simulink model "Plant"  (R2023a)
settings: Solver=VariableStepAuto  StartTime=0.0  StopTime=20  RelTol=1e-3
libraries: slpidlib x2
settings Model: Creator=abhi2  LastModifiedBy=abhi2
settings DebuggingCC: AlgebraicLoopMsg=none

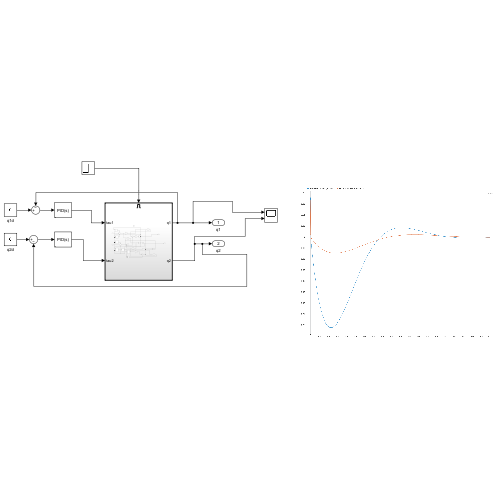
[thumbnail: Simulink's stored preview of the top-level diagram]
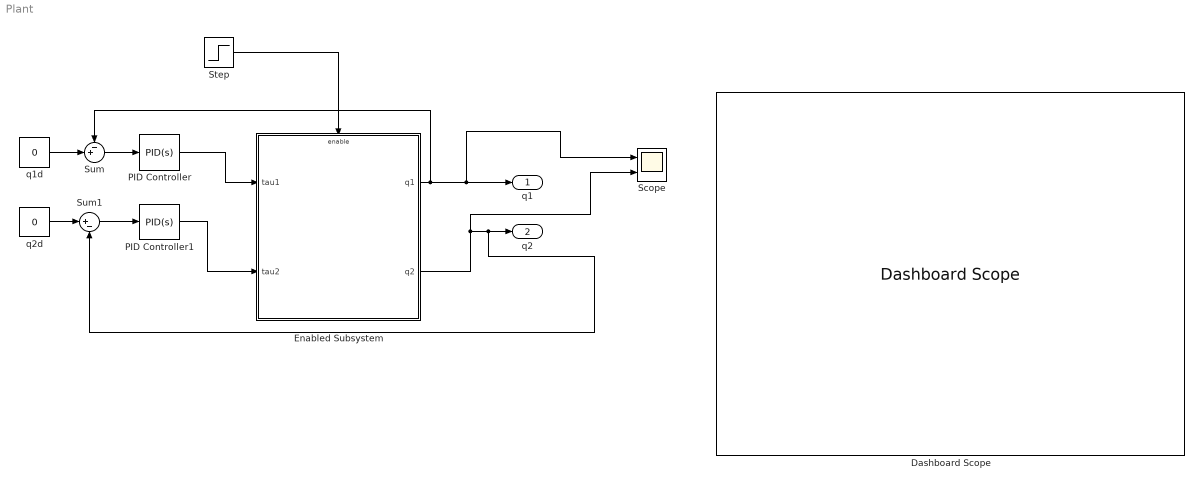
== system Plant ==
  Dashboard Scope : DashboardScope  Ymin=-0.8  Ymax=0.15
  Enabled Subsystem : Subsystem  TreatAsAtomicUnit=on
  PID Controller : slpidlib/PID Controller  Controller=PID  Form=Parallel  TimeDomain=Continuous-time  UseExternalTs=off  SampleTime=-1  IntegratorMethod=Forward Euler  FilterMethod=Forward Euler  ControllerParametersSource=internal  P=80  I=70  UseKiTs=off  D=70  N=1000000  UseFilter=on  TunerSelectOption=Transfer Function Based (PID Tuner App)  InitialConditionSource=internal  InitialConditionForIntegrator=0  InitialConditionForFilter=0  DifferentiatorICPrevScaledInput=0  ExternalReset=none  TrackingMode=off  Kt=1  LimitOutput=off  SatLimitsSource=internal  UpperSaturationLimit=inf  LowerSaturationLimit=-inf  LinearizeAsGain=on  AntiWindupMode=none  Kb=1  LimitIntegrator=off  UpperIntegratorSaturationLimit=inf  LowerIntegratorSaturationLimit=-inf  POutMin=[]  POutMax=[]  IOutMin=[]  IOutMax=[]  DOutMin=[]  DOutMax=[]  NOutMin=[]  NOutMax=[]  SumOutMin=[]  SumOutMax=[]  SaturationOutMin=[]  SaturationOutMax=[]  PParamMin=[]  PParamMax=[]  IParamMin=[]  IParamMax=[]  DParamMin=[]  DParamMax=[]  NParamMin=[]  NParamMax=[]  KbParamMin=[]  KbParamMax=[]  KtParamMin=[]  KtParamMax=[]  KbOutMin=[]  KbOutMax=[]  KtOutMin=[]  KtOutMax=[]  IntegratorOutMin=[]  IntegratorOutMax=[]  FilterOutMin=[]  FilterOutMax=[]  SumI1OutMin=[]  SumI1OutMax=[]  SumI2OutMin=[]  SumI2OutMax=[]  SumI3OutMin=[]  SumI3OutMax=[]  SumI4OutMin=[]  SumI4OutMax=[]  SumDOutMin=[]  SumDOutMax=[]  DifferentiatorOutMin=[]  DifferentiatorOutMax=[]  FilterDiffOutCoefMin=[]  FilterDiffOutCoefMax=[]  ReciprocalOutMin=[]  ReciprocalOutMax=[]  SumDenOutMin=[]  SumDenOutMax=[]  SumNumOutMin=[]  SumNumOutMax=[]  DivideOutMin=[]  DivideOutMax=[]  UdiffTsProdOutMin=[]  UdiffTsProdOutMax=[]  NTsProdOutMin=[]  NTsProdOutMax=[]  UintegralTsProdOutMin=[]  UintegralTsProdOutMax=[]  UngainTsProdOutMin=[]  UngainTsProdOutMax=[]  ClampingZeroOutDataTypeStr=Inherit: Inherit via back propagation  ClampingZeroOutMin=[]  ClampingZeroOutMax=[]  FilterDenConstantOutDataTypeStr=Inherit: Inherit via back propagation  FilterDenConstantOutMin=[]  FilterDenConstantOutMax=[]  PCopyOutDataTypeStr=Inherit: Inherit via back propagation  PCopyOutMin=[]  PCopyOutMax=[]  NCopyOutDataTypeStr=Inherit: Inherit via back propagation  NCopyOutMin=[]  NCopyOutMax=[]  IntegratorContinuousStateAttributes=''  IntegratorStateMustResolveToSignalObject=off  IntegratorRTWStateStorageClass=Auto  FilterContinuousStateAttributes=''  FilterStateMustResolveToSignalObject=off  FilterRTWStateStorageClass=Auto  ParallelPVariant=InternalParameters  IdealPVariant=Disabled  IVariant=InternalParameters  DVariant=InternalParameters  IntegratorVariant=Continuous  SatVariant=Disabled  AWVariant=Passthrough  PCopyVariant=Disabled  TRVariant=Disabled  FdbkBlocksVariant=Forward  IdealPFdbkVariant=Disabled  SatFdbkVariant=Disabled  DerivativeFilterVariant=ContFilter  NVariant=InternalParameters  NCopyVariant=Disabled  FilterICVariant=InternalICsFilter  IntegratorICVariant=InternalICs  ExternalResetVariant=Disabled  TRSumVariant=Passthrough  SumFdbkVariant=Disabled  SumVariant=Sum_PID  TsampFilterVariant=InternalTs  TsampNgainVariant=Passthrough  TsampIntegralVariant=Disabled_SignalSpec  ExternalSaturationOutDataTypeStr=Inherit: Same as second input
  PID Controller1 : slpidlib/PID Controller  Controller=PID  Form=Parallel  TimeDomain=Continuous-time  UseExternalTs=off  SampleTime=-1  IntegratorMethod=Forward Euler  FilterMethod=Forward Euler  ControllerParametersSource=internal  P=60  I=50  UseKiTs=off  D=70  N=1000000  UseFilter=on  TunerSelectOption=Transfer Function Based (PID Tuner App)  InitialConditionSource=internal  InitialConditionForIntegrator=0  InitialConditionForFilter=0  DifferentiatorICPrevScaledInput=0  ExternalReset=none  TrackingMode=off  Kt=1  LimitOutput=off  SatLimitsSource=internal  UpperSaturationLimit=inf  LowerSaturationLimit=-inf  LinearizeAsGain=on  AntiWindupMode=none  Kb=1  LimitIntegrator=off  UpperIntegratorSaturationLimit=inf  LowerIntegratorSaturationLimit=-inf  POutMin=[]  POutMax=[]  IOutMin=[]  IOutMax=[]  DOutMin=[]  DOutMax=[]  NOutMin=[]  NOutMax=[]  SumOutMin=[]  SumOutMax=[]  SaturationOutMin=[]  SaturationOutMax=[]  PParamMin=[]  PParamMax=[]  IParamMin=[]  IParamMax=[]  DParamMin=[]  DParamMax=[]  NParamMin=[]  NParamMax=[]  KbParamMin=[]  KbParamMax=[]  KtParamMin=[]  KtParamMax=[]  KbOutMin=[]  KbOutMax=[]  KtOutMin=[]  KtOutMax=[]  IntegratorOutMin=[]  IntegratorOutMax=[]  FilterOutMin=[]  FilterOutMax=[]  SumI1OutMin=[]  SumI1OutMax=[]  SumI2OutMin=[]  SumI2OutMax=[]  SumI3OutMin=[]  SumI3OutMax=[]  SumI4OutMin=[]  SumI4OutMax=[]  SumDOutMin=[]  SumDOutMax=[]  DifferentiatorOutMin=[]  DifferentiatorOutMax=[]  FilterDiffOutCoefMin=[]  FilterDiffOutCoefMax=[]  ReciprocalOutMin=[]  ReciprocalOutMax=[]  SumDenOutMin=[]  SumDenOutMax=[]  SumNumOutMin=[]  SumNumOutMax=[]  DivideOutMin=[]  DivideOutMax=[]  UdiffTsProdOutMin=[]  UdiffTsProdOutMax=[]  NTsProdOutMin=[]  NTsProdOutMax=[]  UintegralTsProdOutMin=[]  UintegralTsProdOutMax=[]  UngainTsProdOutMin=[]  UngainTsProdOutMax=[]  ClampingZeroOutDataTypeStr=Inherit: Inherit via back propagation  ClampingZeroOutMin=[]  ClampingZeroOutMax=[]  FilterDenConstantOutDataTypeStr=Inherit: Inherit via back propagation  FilterDenConstantOutMin=[]  FilterDenConstantOutMax=[]  PCopyOutDataTypeStr=Inherit: Inherit via back propagation  PCopyOutMin=[]  PCopyOutMax=[]  NCopyOutDataTypeStr=Inherit: Inherit via back propagation  NCopyOutMin=[]  NCopyOutMax=[]  IntegratorContinuousStateAttributes=''  IntegratorStateMustResolveToSignalObject=off  IntegratorRTWStateStorageClass=Auto  FilterContinuousStateAttributes=''  FilterStateMustResolveToSignalObject=off  FilterRTWStateStorageClass=Auto  ParallelPVariant=InternalParameters  IdealPVariant=Disabled  IVariant=InternalParameters  DVariant=InternalParameters  IntegratorVariant=Continuous  SatVariant=Disabled  AWVariant=Passthrough  PCopyVariant=Disabled  TRVariant=Disabled  FdbkBlocksVariant=Forward  IdealPFdbkVariant=Disabled  SatFdbkVariant=Disabled  DerivativeFilterVariant=ContFilter  NVariant=InternalParameters  NCopyVariant=Disabled  FilterICVariant=InternalICsFilter  IntegratorICVariant=InternalICs  ExternalResetVariant=Disabled  TRSumVariant=Passthrough  SumFdbkVariant=Disabled  SumVariant=Sum_PID  TsampFilterVariant=InternalTs  TsampNgainVariant=Passthrough  TsampIntegralVariant=Disabled_SignalSpec  ExternalSaturationOutDataTypeStr=Inherit: Same as second input
  Scope : Scope  NumInputPorts=2
  Step : Step  Time=0  SampleTime=0
  Sum : Sum  Inputs=-+|
  Sum1 : Sum  Inputs=|+-
  q1d : Constant  Value=0
  q2d : Constant  Value=0
  q1 : Outport
  q2 : Outport  Port=2
  wires:
  Enabled Subsystem/2(q2) -> Scope/2, Sum1/2, q2/1
  q2d/1 -> Sum1/1
  Sum1/1 -> PID Controller1/1
  q1d/1 -> Sum/2
  PID Controller1/1 -> Enabled Subsystem/2(tau2)
  Sum/1 -> PID Controller/1
  PID Controller/1 -> Enabled Subsystem/1(tau1)
  Enabled Subsystem/1(q1) -> Sum/1, Scope/1, q1/1
  Step/1 -> Enabled Subsystem/Enable

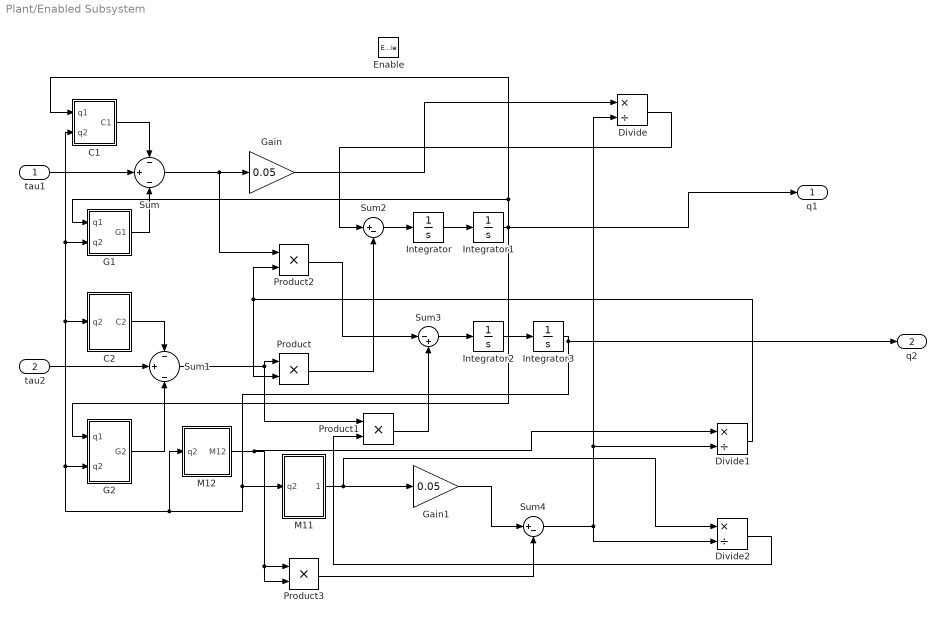
== system Plant/Enabled Subsystem ==
  tau1 : Inport
  tau2 : Inport  Port=2
  Enable : EnablePort
  C1 : Subsystem
  C2 : Subsystem
  Divide : Product  Inputs=*/
  Divide1 : Product  Inputs=*/
  Divide2 : Product  Inputs=*/
  G1 : Subsystem
  G2 : Subsystem
  Gain : Gain  Gain=0.05
  Gain1 : Gain  Gain=0.05
  Integrator : Integrator
  Integrator1 : Integrator  InitialCondition=0.1
  Integrator2 : Integrator
  Integrator3 : Integrator  InitialCondition=0.1
  M11 : Subsystem
  M12 : Subsystem
  Product{,1..3} (4 alike) : Product
  Sum : Sum  Inputs=-|+|-
  Sum1 : Sum  Inputs=-|+|-
  Sum2 : Sum  Inputs=|+-
  Sum3 : Sum  Inputs=|-+
  Sum4 : Sum  Inputs=|+-
  q1 : Outport  SourceOfInitialOutputValue=Input signal  OutputWhenDisabled=reset  InitialOutput=[0.1]
  q2 : Outport  Port=2  SourceOfInitialOutputValue=Input signal  OutputWhenDisabled=reset  InitialOutput=[0.1]
  wires:
  Integrator/1 -> Integrator1/1
  tau2/1 -> Sum1/2
  C2/1(C2) -> Sum1/1
  Sum/1 -> Gain/1, Product2/1
  M12/1(M12) -> Product3/2, Product3/1, Divide1/1
  Sum3/1 -> Integrator2/1
  Sum2/1 -> Integrator/1
  Product/1 -> Sum2/2
  Sum1/1 -> Product/1, Product1/1
  Product1/1 -> Sum3/2
  G2/1(G2) -> Sum1/3
  Product2/1 -> Sum3/1
  G1/1(G1) -> Sum/3
  Integrator2/1 -> Integrator3/1
  C1/1(C1) -> Sum/1
  tau1/1 -> Sum/2
  Gain/1 -> Divide/1
  M11/1(M11) -> Divide2/1, Gain1/1
  Gain1/1 -> Sum4/1
  Product3/1 -> Sum4/2
  Sum4/1 -> Divide2/2, Divide1/2, Divide/2
  Divide/1 -> Sum2/1
  Divide1/1 -> Product/2, Product2/2
  Divide2/1 -> Product1/2
  Integrator1/1 -> q1/1, G2/1(q1), G1/1(q1), C1/1(q1)
  Integrator3/1 -> q2/1, C1/2(q2), G1/2(q2), C2/1(q2), G2/2(q2), M12/1(q2), M11/1(q2)

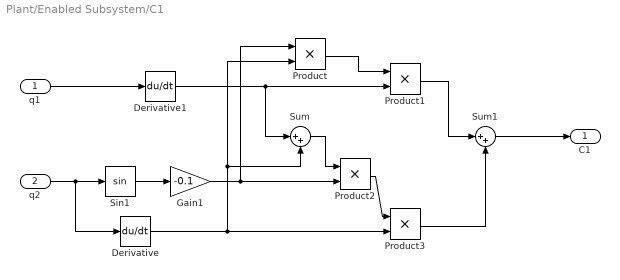
== system Plant/Enabled Subsystem/C1 ==
  q1 : Inport
  q2 : Inport  Port=2
  Derivative : Derivative
  Derivative1 : Derivative
  Gain1 : Gain  Gain=-0.1
  Product{,1..3} (4 alike) : Product
  Sin1 : Trigonometry
  Sum : Sum  Inputs=|++
  Sum1 : Sum  Inputs=|++
  C1 : Outport
  wires:
  Product1/1 -> Sum1/1
  Derivative/1 -> Product3/2, Sum/2, Product/2
  q1/1 -> Derivative1/1
  Sum/1 -> Product2/1
  Product/1 -> Product1/1
  Gain1/1 -> Product/1, Product2/2
  Product2/1 -> Product3/1
  Derivative1/1 -> Sum/1, Product1/2
  Product3/1 -> Sum1/2
  Sin1/1 -> Gain1/1
  q2/1 -> Derivative/1, Sin1/1
  Sum1/1 -> C1/1

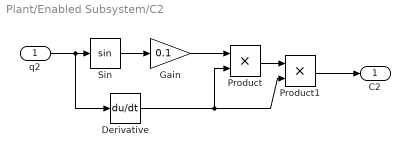
== system Plant/Enabled Subsystem/C2 ==
  q2 : Inport
  Derivative : Derivative
  Gain : Gain  Gain=0.1
  Product : Product
  Product1 : Product
  Sin : Trigonometry
  C2 : Outport
  wires:
  Sin/1 -> Gain/1
  Derivative/1 -> Product1/2, Product/2
  q2/1 -> Derivative/1, Sin/1
  Product1/1 -> C2/1
  Product/1 -> Product1/1
  Gain/1 -> Product/1

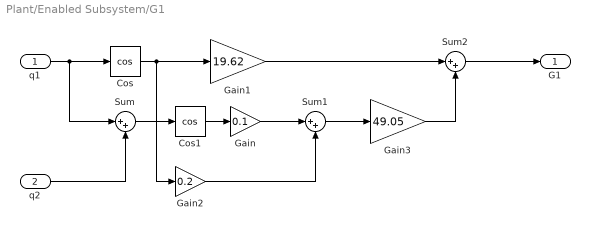
== system Plant/Enabled Subsystem/G1 ==
  q1 : Inport
  q2 : Inport  Port=2
  Cos : Trigonometry  Operator=cos
  Cos1 : Trigonometry  Operator=cos
  Gain : Gain  Gain=0.1
  Gain1 : Gain  Gain=19.62
  Gain2 : Gain  Gain=0.2
  Gain3 : Gain  Gain=49.05
  Sum : Sum  Inputs=|++
  Sum1 : Sum  Inputs=|++
  Sum2 : Sum  Inputs=|++
  G1 : Outport
  wires:
  Gain/1 -> Sum1/1
  Sum/1 -> Cos1/1
  Cos/1 -> Gain2/1, Gain1/1
  Cos1/1 -> Gain/1
  q1/1 -> Sum/1, Cos/1
  Gain1/1 -> Sum2/1
  Sum2/1 -> G1/1
  q2/1 -> Sum/2
  Gain2/1 -> Sum1/2
  Sum1/1 -> Gain3/1
  Gain3/1 -> Sum2/2

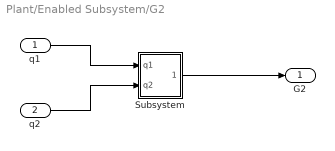
== system Plant/Enabled Subsystem/G2 ==
  q1 : Inport
  q2 : Inport  Port=2
  Subsystem : Subsystem
  G2 : Outport
  wires:
  Subsystem/1(Output) -> G2/1
  q2/1 -> Subsystem/2(q2)
  q1/1 -> Subsystem/1(q1)

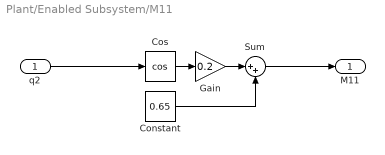
== system Plant/Enabled Subsystem/M11 ==
  q2 : Inport
  Constant : Constant  Value=0.65
  Cos : Trigonometry  Operator=cos
  Gain : Gain  Gain=0.2
  Sum : Sum  Inputs=|++
  M11 : Outport
  wires:
  Gain/1 -> Sum/1
  Cos/1 -> Gain/1
  q2/1 -> Cos/1
  Constant/1 -> Sum/2
  Sum/1 -> M11/1

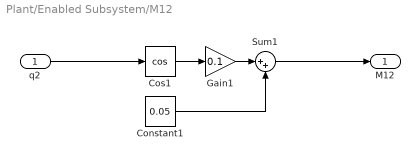
== system Plant/Enabled Subsystem/M12 ==
  q2 : Inport
  Constant1 : Constant  Value=0.05
  Cos1 : Trigonometry  Operator=cos
  Gain1 : Gain  Gain=0.1
  Sum1 : Sum  Inputs=|++
  M12 : Outport
  wires:
  Constant1/1 -> Sum1/2
  Sum1/1 -> M12/1
  Cos1/1 -> Gain1/1
  Gain1/1 -> Sum1/1
  q2/1 -> Cos1/1

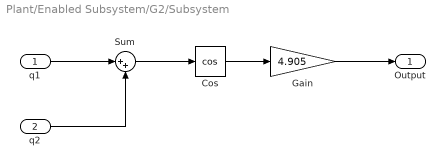
== system Plant/Enabled Subsystem/G2/Subsystem ==
  q1 : Inport
  q2 : Inport  Port=2
  Cos : Trigonometry  Operator=cos
  Gain : Gain  Gain=4.905
  Sum : Sum  Inputs=|++
  Output : Outport
  wires:
  q2/1 -> Sum/2
  q1/1 -> Sum/1
  Sum/1 -> Cos/1
  Cos/1 -> Gain/1
  Gain/1 -> Output/1
